simulink model "cau52b"  (R2015a)
settings: Solver=ode3  StartTime=0.0  StopTime=10.0  RelTol=1e-3
libraries: commfilt2 x4, dspsrcs4 x4, dspstat3 x1, commchan3 x1, commsink2 x1, commutil2 x1, commanapbnd3 x1, commrandsrc2 x1
settings Model: Creator=Ming Duc  LastModifiedBy=Admin
settings DataIOCC: LoadExternalInput=on

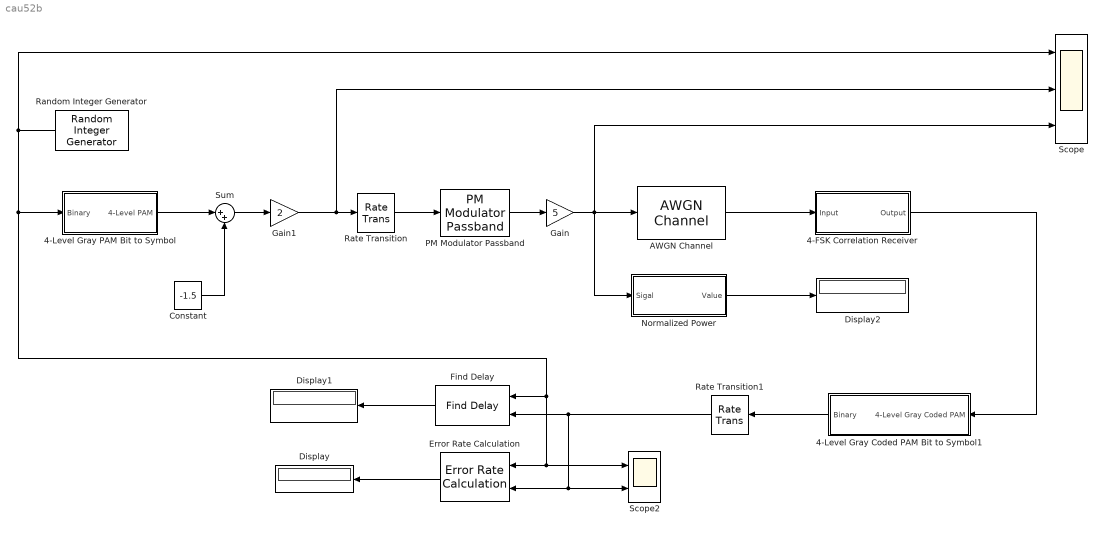
== system cau52b ==
  " Normalized Power" : Subsystem
  4-FSK Correlation Receiver : Subsystem
  4-Level Gray Coded PAM Bit to Symbol1 : Subsystem
  4-Level Gray PAM Bit to Symbol : Subsystem
  AWGN Channel : commchan3/AWGN Channel  InputProcessing=Columns as channels (frame based)  seed=67  noiseMode="Signal to noise ratio  (Eb/No)"  EbNodB=6  EsNodB=10  SNRdB=10  bitsPerSym=1  Ps=1  Tsym=1  variance=1
  Constant : Constant  Value=-1.5
  Display : Display
  Display1 : Display
  Display2 : Display
  Error Rate Calculation : commsink2/Error Rate Calculation  N=0  st_delay=0  cp_mode=Select samples from mask  subframe=1  PMode=Port  WsName=ErrorVec  RsMode2=off  stop=off  numErr=100  maxBits=1e6
  Find Delay : commutil2/Find Delay  corrLength=200  chgSigOP=off  stopUpdate=off  numConstDelay=3
  Gain : Gain  Gain=5
  Gain1 : Gain  Gain=2
  PM Modulator Passband : commanapbnd3/PM Modulator Passband  Fc=300  Ph=0  Kc=pi/2
  Random Integer Generator : commrandsrc2/Random Integer Generator  mul=2  seed=37  Ts=1e-5  frameBased=off  sampPerFrame=1  orient=off  outDataType=double
  Rate Transition : RateTransition  OutPortSampleTime=2e-5
  Rate Transition1 : RateTransition  OutPortSampleTime=1/1000
  Scope : Scope  NumInputPorts=3
      settings: YMin=-5~-5~-5  YMax=5~5~5
  Scope2 : Scope  NumInputPorts=2
      settings: YMin=-5~-5  YMax=5~5  SaveName=ScopeData2
  Sum : Sum  Inputs=|++
  wires:
  Random Integer Generator/1 -> Scope/1, Find Delay/1, Scope2/1, Error Rate Calculation/1, 4-Level Gray PAM Bit to Symbol/1(Binary)
  Rate Transition1/1 -> Error Rate Calculation/2, Scope2/2, Find Delay/2
  4-Level Gray Coded PAM Bit to Symbol1/1(Binary) -> Rate Transition1/1
  Rate Transition/1 -> PM Modulator Passband/1
  PM Modulator Passband/1 -> Gain/1
  Gain/1 -> " Normalized Power"/1(Sigal), Scope/3, AWGN Channel/1
  Find Delay/1 -> Display1/1
  Error Rate Calculation/1 -> Display/1
  " Normalized Power"/1(Value) -> Display2/1
  AWGN Channel/1 -> 4-FSK Correlation Receiver/1(Input)
  4-FSK Correlation Receiver/1(Output) -> 4-Level Gray Coded PAM Bit to Symbol1/1(4-Level Gray Coded PAM)
  Sum/1 -> Gain1/1
  Constant/1 -> Sum/2
  4-Level Gray PAM Bit to Symbol/1(4-Level PAM) -> Sum/1
  Gain1/1 -> Scope/2, Rate Transition/1

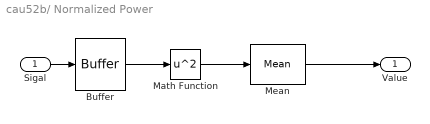
== system cau52b/ Normalized Power ==
  Sigal : Inport
  Buffer : Buffer  TreatMby1Signals=One channel
  Math Function : Math  Operator=square  SaturateOnIntegerOverflow=on
  Mean : dspstat3/Mean  run=off  reset_popup=None  InputProcessing=Columns as channels (frame based)  directionMode=Each column  dimension=1  treatSBRowAsCol=off  roiEnable=off  roiType=Rectangles  roiPortion=Entire ROI  roiOutput=Individual statistics for each ROI  roiFlag=off  outputDataTypeStr=Inherit: Same as accumulator  outputLastDataTypeStr=Inherit: Same as accumulator  outputMin=[]  outputMax=[]  roundingMode=Floor  overflowMode=off
  Value : Outport
  wires:
  Sigal/1 -> Buffer/1
  Buffer/1 -> Math Function/1
  Math Function/1 -> Mean/1
  Mean/1 -> Value/1

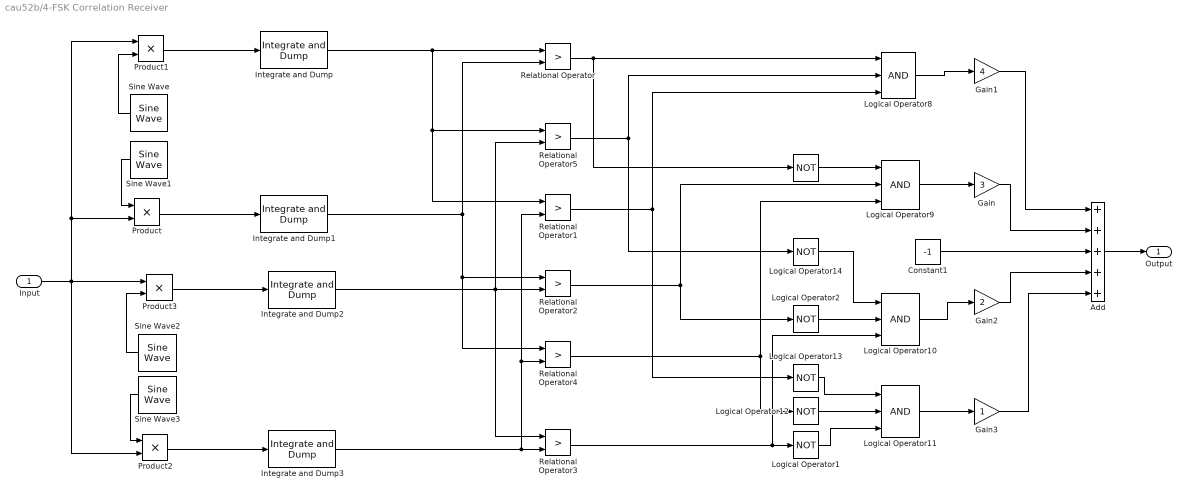
== system cau52b/4-FSK Correlation Receiver ==
  Input : Inport
  " " : Logic  Operator=NOT  IconShape=distinctive  AllPortsSameDT=off  OutDataTypeStr=boolean
  Add : Sum  Inputs=+++++
  Constant1 : Constant  Value=-1
  Gain : Gain  Gain=3
  Gain1 : Gain  Gain=4
  Gain2 : Gain  Gain=2
  Gain3 : Gain
  Integrate and Dump{,1..3} (4 alike) : commfilt2/Integrate and Dump  obssamples=8  offsetsamples=0  nodump=off  roundingMode=Floor  overflowMode=off
  Logical Operator{1..2,12..14} (5 alike) : Logic  Operator=NOT  IconShape=distinctive  AllPortsSameDT=off  OutDataTypeStr=boolean
  Logical Operator{8..11} (4 alike) : Logic  Inputs=3  AllPortsSameDT=off  OutDataTypeStr=boolean
  Product{,1..3} (4 alike) : Product
  Relational Operator{,1..5} (6 alike) : RelationalOperator  Operator=>  OutDataTypeStr=boolean
  Sine Wave{,1..3} (4 alike) : dspsrcs4/Sine Wave  Amplitude=1  Frequency=100  Phase=0  SampleMode=Discrete  OutComplex=Real  CompMethod=Trigonometric fcn  TableSize=Speed  SampleTime=1/1000  SamplesPerFrame=1  ResetState=Restart at time zero  dataType=double  wordLen=16  udDataType=sfix(16)  fracBitsMode=Best precision  numFracBits=15  OutDataTypeStr=double  LastOutDataTypeStr=double
  Output : Outport
  wires:
  Sine Wave1/1 -> Product/1
  Sine Wave/1 -> Product1/2
  Product1/1 -> Integrate and Dump/1
  Integrate and Dump/1 -> Relational Operator/1, Relational Operator5/1, Relational Operator1/1
  Product/1 -> Integrate and Dump1/1
  Add/1 -> Output/1
  Gain3/1 -> Add/5
  Gain2/1 -> Add/4
  Constant1/1 -> Add/3
  Gain/1 -> Add/2
  Gain1/1 -> Add/1
  Sine Wave3/1 -> Product2/1
  Sine Wave2/1 -> Product3/2
  Product3/1 -> Integrate and Dump2/1
  Integrate and Dump2/1 -> Relational Operator2/2, Relational Operator3/1, Relational Operator5/2
  Product2/1 -> Integrate and Dump3/1
  Input/1 -> Product1/1, Product/2, Product2/2, Product3/1
  Logical Operator8/1 -> Gain1/1
  Logical Operator9/1 -> Gain/1
  Logical Operator10/1 -> Gain2/1
  Logical Operator11/1 -> Gain3/1
  Logical Operator1/1 -> Logical Operator11/3
  Logical Operator12/1 -> Logical Operator11/2
  Logical Operator13/1 -> Logical Operator11/1
  Logical Operator2/1 -> Logical Operator10/2
  Logical Operator14/1 -> Logical Operator10/1
  Relational Operator3/1 -> Logical Operator1/1, Logical Operator10/3
  " "/1 -> Logical Operator9/1
  Relational Operator/1 -> Logical Operator8/1, " "/1
  Integrate and Dump1/1 -> Relational Operator/2, Relational Operator2/1, Relational Operator4/1
  Integrate and Dump3/1 -> Relational Operator4/2, Relational Operator1/2, Relational Operator3/2
  Relational Operator4/1 -> Logical Operator12/1, Logical Operator9/3
  Relational Operator1/1 -> Logical Operator8/3, Logical Operator13/1
  Relational Operator5/1 -> Logical Operator14/1, Logical Operator8/2
  Relational Operator2/1 -> Logical Operator9/2, Logical Operator2/1

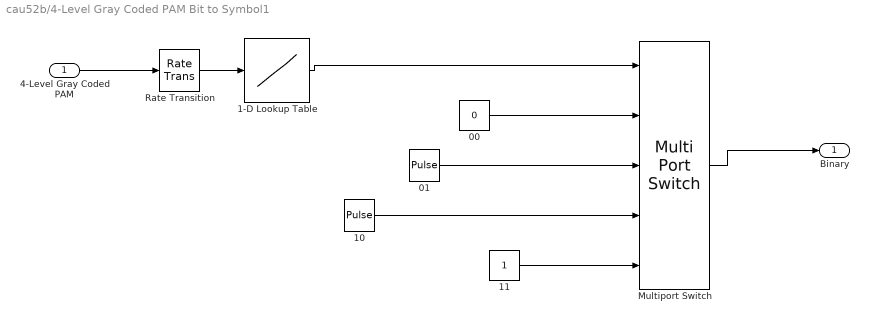
== system cau52b/4-Level Gray Coded PAM Bit to Symbol1 ==
  4-Level Gray Coded PAM : Inport
  00 : Constant  Value=0
  01 : DiscretePulseGenerator  Amplitude=4  Period=10  PulseWidth=5  SampleTime=1/1000
  1-D Lookup Table : Lookup_n-D  NumberOfTableDimensions=1  BreakpointsForDimension1=[-5:5]  Table=tanh([-5:5])  InternalRulePriority=Speed  RndMeth=Simplest  InputSameDT=on
  10 : DiscretePulseGenerator  Amplitude=4  Period=10  PulseWidth=5  PhaseDelay=2  SampleTime=1/1000
  11 : Constant
  Multiport Switch : MultiPortSwitch  Inputs=4  DiagnosticForDefault=None
  Rate Transition : RateTransition
  Binary : Outport
  wires:
  4-Level Gray Coded PAM/1 -> Rate Transition/1
  Multiport Switch/1 -> Binary/1
  Rate Transition/1 -> 1-D Lookup Table/1
  1-D Lookup Table/1 -> Multiport Switch/1
  00/1 -> Multiport Switch/2
  01/1 -> Multiport Switch/3
  10/1 -> Multiport Switch/4
  11/1 -> Multiport Switch/5

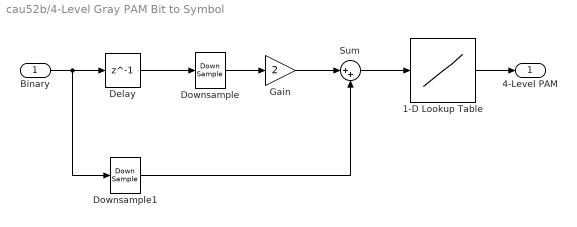
== system cau52b/4-Level Gray PAM Bit to Symbol ==
  Binary : Inport
  1-D Lookup Table : Lookup_n-D  NumberOfTableDimensions=1  BreakpointsForDimension1=[1,2,3]  Table=[0,4,2]  InternalRulePriority=Speed  RndMeth=Simplest  InputSameDT=on
  Delay : Delay  DelayLength=1  InitialCondition=0
  Downsample : DownSample  RateOptions=Allow multirate processing
  Downsample1 : DownSample  RateOptions=Allow multirate processing
  Gain : Gain  Gain=2
  Sum : Sum  Inputs=|++
  4-Level PAM : Outport
  wires:
  Sum/1 -> 1-D Lookup Table/1
  1-D Lookup Table/1 -> 4-Level PAM/1
  Binary/1 -> Downsample1/1, Delay/1
  Delay/1 -> Downsample/1
  Downsample/1 -> Gain/1
  Gain/1 -> Sum/1
  Downsample1/1 -> Sum/2
